simulink model "DSX_serial_sending_1"  (R2020b)
settings: Solver=FixedStepAuto  StartTime=0.0  StopTime=inf  RelTol=1e-3
model workspace (MAT data in the model file):
  NOT_CONSTANT = 3.16513761468
  Period = 1
  STRING_VALUE = "fast"
  device = "device"
  func = "func"
  port = "port"
  value = "value"
undefined symbols (not defined in the file): LF, serial
libraries: instrumentlib x3, sldrtlib x1
settings Model: FPTRunName=Active  SILPILModeSetting=veronly  ExtModeTrigDuration=2  Creator=16047  LastModifiedBy=16047
settings DataIOCC: LimitDataPoints=on  SaveFormat=Array
settings OptimizationCC: ExpressionDepthLimit=2147483647  LifeSpan=Inf  MaxStackSize=64
settings DebuggingCC: UnderspecifiedInitializationDetection=Classic  MergeDetectMultiDrivingBlocksExec=none  FcnCallInpInsideContextMsg=warning  AllowSymbolicDim=off  StateNameClashWarn=warning  SFUnexpectedBacktrackingDiag=warning  SFNoUnconditionalDefaultTransitionDiag=warning  SFExecutionAtInitializationDiag=none  ArithmeticOperatorsInVariantConditions=warning
settings HardwareCC: ProdBitPerInt=16  ProdBitPerPointer=16  ProdBitPerSizeT=16  ProdBitPerPtrDiffT=16  ProdLargestAtomicFloat=None  ProdWordSize=8  ProdHWDeviceType=Atmel->AVR
settings ModelReferenceCC: PropagateSignalLabelsOutOfModel=off
settings SFSimCC: SimUseLocalCustomCode=off  CustomCodeUndefinedFunction=UseInterfaceOnly
settings RTWCC: Description=Embedded Coder  SystemTargetFile=ert.tlc  HardwareBoard=Arduino Uno  TemplateMakefile=ert_default_tmf  GenerateReport=on  RTWVerbose=off  RTWUseLocalCustomCode=off  Toolchain=Arduino AVR  BuildConfiguration=Faster Runs  LaunchReport=on
settings CodeAppCC: ForceParamTrailComments=on  OperatorAnnotations=on  StateflowObjectComments=on  MATLABSourceComments=on
settings ERTTargetCC: MultiwordLength=2048  ERTCustomFileBanners=off  SupportContinuousTime=on  SupportNonInlinedSFcns=on  RemoveResetFunc=off  SupportVariableSizeSignals=on  ModelStepFunctionPrototypeControlCompliant=off  ExtModeStaticAllocSize=250
settings ConfigComp: CovMetricSettings=dw  CovSaveCumulativeToWorkspaceVar=on  CovSaveSingleToWorkspaceVar=on  CovExternalEMLEnable=off  CovSFcnEnable=off

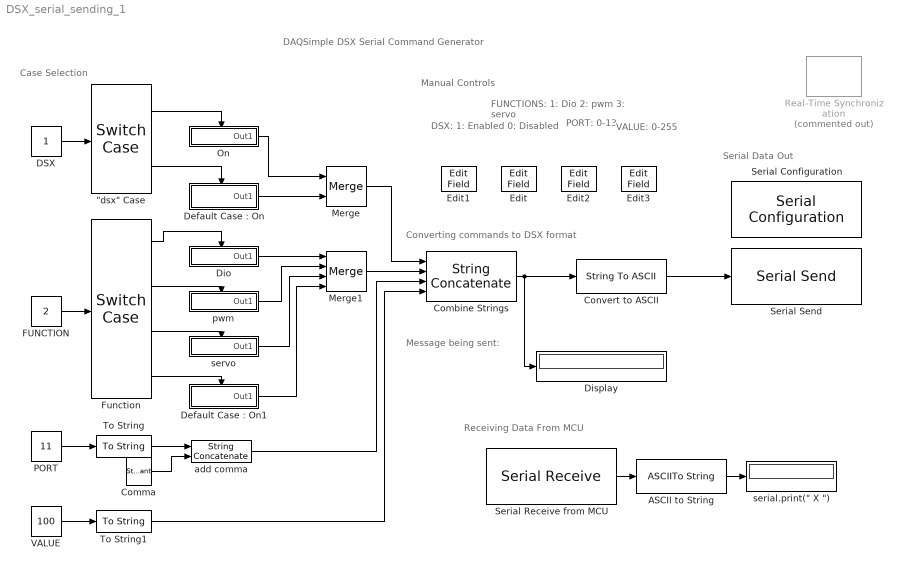
== system DSX_serial_sending_1 ==
  note: Message being sent:
  note: DAQSimple DSX Serial Command Generator
  note: Converting commands to DSX format
  note: Receiving Data From MCU
  note: Case Selection
  note: Serial Data Out
  note: Manual Controls
  note: FUNCTIONS:
      | 1: Dio
      | 2: pwm
      | 3: servo
  note: DSX:
      | 1: Enabled
      | 0: Disabled
  note: PORT:
      | 0-13
  note: VALUE:
      | 0-255
  "\"dsx\" Case" : SwitchCase
  ASCII to String : ASCIIToString
  Combine Strings : StringConcatenate  Inputs=4
  Comma : StringConstant  String="\",\""
  Convert to ASCII : StringToASCII
  DSX : Constant
  "Default Case : On" : Subsystem  TreatAsAtomicUnit=on
  "Default Case : On1" : Subsystem  TreatAsAtomicUnit=on
  Dio : Subsystem  TreatAsAtomicUnit=on
  Display : Display
      settings: Format=bank
  Edit{,1..3} (4 alike) : EditField  LabelPosition=Hide  ShowInitialText=on  Alignment=Center
  FUNCTION : Constant  Value=2
  Function : SwitchCase  CaseConditions={1,2,3}
  Merge : Merge
  Merge1 : Merge  Inputs=4
  On : Subsystem  TreatAsAtomicUnit=on
  PORT : Constant  Value=11
  Real-Time Synchronization : sldrtlib/Real-Time Synchronization  Commented=on  SampleTime=0.1  MaxMissedTicks=10  ShowMissedTicks=off  YieldWhenWaiting=off
  Serial Configuration : instrumentlib/Serial Configuration  Priority=-200000  ComPortMenu=COM5  ComPort=COM5  ObjConstructor=serial('COM5');  BaudRate=9600  DataBits=8  Parity=none  StopBits=1  FlowControl=none  Timeout=10  ByteOrder=LittleEndian
  Serial Receive from MCU : instrumentlib/Serial Receive  ComPortMenu=<Please select a port...>  ComPort=COM5  ObjConstructor=serial('COM5');  Terminator=LF ('\n')  DataSize=[1 1]  DataType=uint8  EnableBlockingMode=on  ActionDataUnavailable=Output last received value  CustomValue=0  SampleTime=0.01
  Serial Send : instrumentlib/Serial Send  ComPortMenu=COM5  ComPort=COM5  ObjConstructor=serial('COM5');  Terminator=LF ('\n')  EnableBlockingMode=on
  To String : ToString
  To String1 : ToString
  VALUE : Constant  Value=100
  add comma : StringConcatenate
  pwm : Subsystem  TreatAsAtomicUnit=on
  "serial.print(\" X \")" : Display
  servo : Subsystem  TreatAsAtomicUnit=on
  wires:
  Convert to ASCII/1 -> Serial Send/1
  Combine Strings/1 -> Convert to ASCII/1, Display/1
  Serial Receive from MCU/1 -> ASCII to String/1
  ASCII to String/1 -> "serial.print(\" X \")"/1
  DSX/1 -> "\"dsx\" Case"/1
  "\"dsx\" Case"/1 -> On/Action
  On/1(Out1) -> Merge/1
  "\"dsx\" Case"/2 -> "Default Case : On"/Action
  "Default Case : On"/1(Out1) -> Merge/2
  "Default Case : On1"/1(Out1) -> Merge1/4
  Function/4 -> "Default Case : On1"/Action
  Dio/1(Out1) -> Merge1/1
  Function/1 -> Dio/Action
  FUNCTION/1 -> Function/1
  Function/2 -> pwm/Action
  Function/3 -> servo/Action
  servo/1(Out1) -> Merge1/3
  pwm/1(Out1) -> Merge1/2
  PORT/1 -> To String/1
  VALUE/1 -> To String1/1
  Merge/1 -> Combine Strings/1
  Merge1/1 -> Combine Strings/2
  To String1/1 -> Combine Strings/4
  To String/1 -> add comma/1
  add comma/1 -> Combine Strings/3
  Comma/1 -> add comma/2

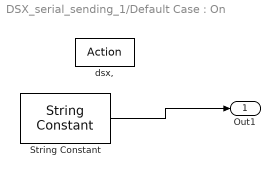
== system DSX_serial_sending_1/Default Case : On ==
  dsx, : ActionPort  ActionPortLabel=default:
  String Constant : StringConstant  String="\"dis,\""
  Out1 : Outport
  wires:
  String Constant/1 -> Out1/1

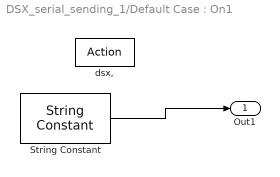
== system DSX_serial_sending_1/Default Case : On1 ==
  dsx, : ActionPort  ActionPortLabel=default:
  String Constant : StringConstant  String="\"def,\""
  Out1 : Outport
  wires:
  String Constant/1 -> Out1/1

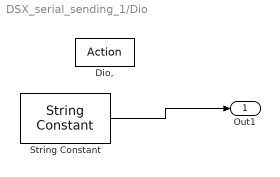
== system DSX_serial_sending_1/Dio ==
  Dio, : ActionPort  ActionPortLabel=case [ 1 ]:
  String Constant : StringConstant  String="\"Dio,\""
  Out1 : Outport
  wires:
  String Constant/1 -> Out1/1

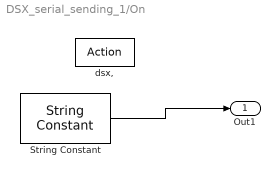
== system DSX_serial_sending_1/On ==
  dsx, : ActionPort  ActionPortLabel=case [ 1 ]:
  String Constant : StringConstant  String="\"dsx,\""
  Out1 : Outport
  wires:
  String Constant/1 -> Out1/1

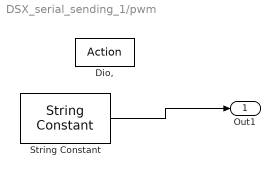
== system DSX_serial_sending_1/pwm ==
  Dio, : ActionPort  ActionPortLabel=case [ 2 ]:
  String Constant : StringConstant  String="\"pwm,\""
  Out1 : Outport
  wires:
  String Constant/1 -> Out1/1

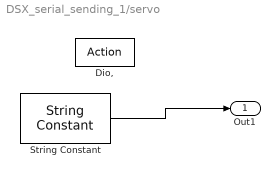
== system DSX_serial_sending_1/servo ==
  Dio, : ActionPort  ActionPortLabel=case [ 3 ]:
  String Constant : StringConstant  String="\"servo,\""
  Out1 : Outport
  wires:
  String Constant/1 -> Out1/1
